simulink model "bai4thuchanh"  (R2016a)
settings: Solver=VariableStepAuto  StartTime=0.0  StopTime=1  RelTol=1e-3
undefined symbols (not defined in the file or in its folder): magnitude
settings Model: Creator=HP  LastModifiedBy=HP

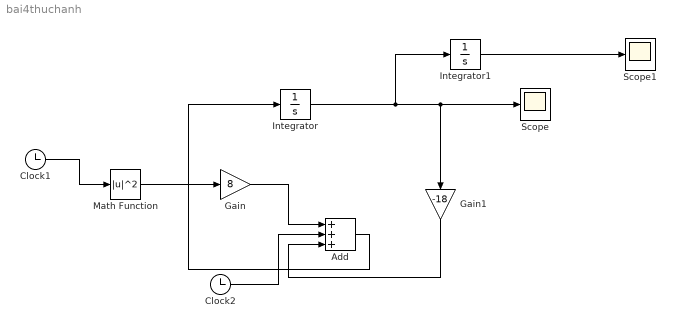
== system bai4thuchanh ==
  Add : Sum  Inputs=+++
  Clock1 : Clock
  Clock2 : Clock
  Gain : Gain  Gain=8
  Gain1 : Gain  Gain=-18
  Integrator : Integrator
  Integrator1 : Integrator
  Math Function : Math  Operator=magnitude^2  SaturateOnIntegerOverflow=on
  Scope : Scope
  Scope1 : Scope
  wires:
  Gain/1 -> Add/1
  Clock2/1 -> Add/2
  Gain1/1 -> Add/3
  Add/1 -> Integrator/1
  Integrator/1 -> Integrator1/1, Gain1/1, Scope/1
  Math Function/1 -> Gain/1
  Clock1/1 -> Math Function/1
  Integrator1/1 -> Scope1/1
